simulink model "X_and_Y_position_calculator_of_the_center_of_mass_of_a_car"  (R2022b)
settings: Solver=VariableStepAuto  StartTime=0.0  StopTime=10.0  RelTol=1e-3
settings Model: Creator=tom  LastModifiedBy=tom

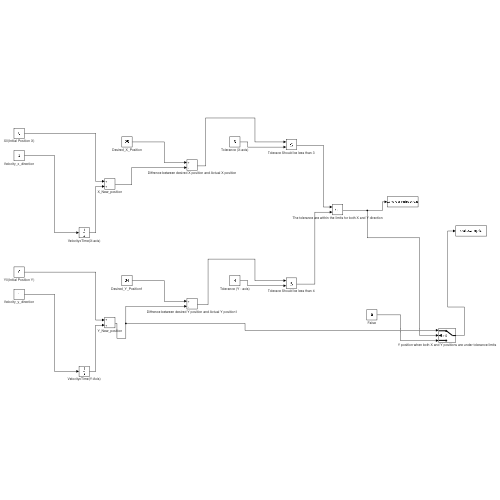
[thumbnail: Simulink's stored preview of the top-level diagram]
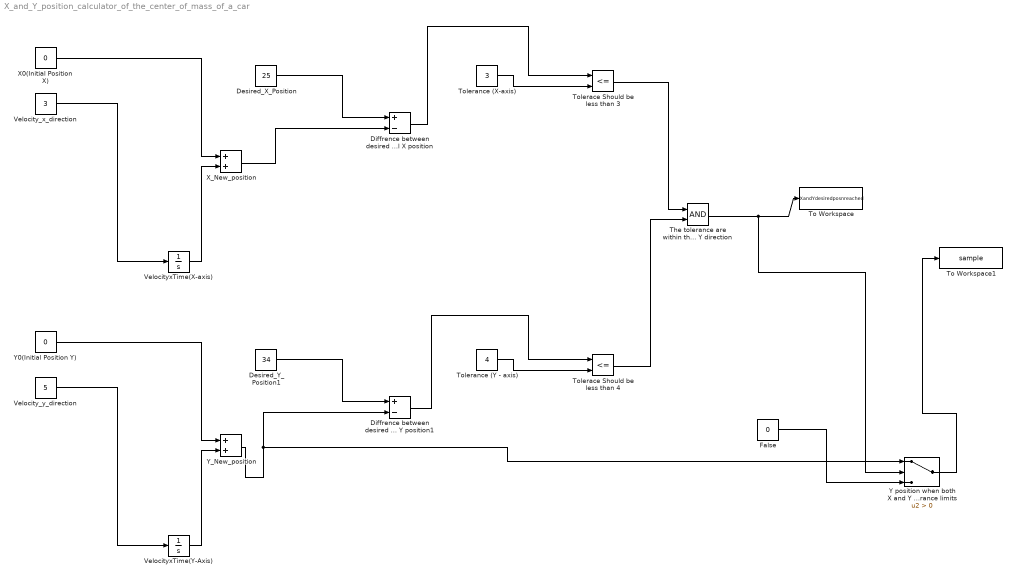
== system X_and_Y_position_calculator_of_the_center_of_mass_of_a_car ==
  Desired_X_Position : Constant  Value=25
  Desired_Y_Position1 : Constant  Value=34
  Diffrence between desired X position and Actual X position : Sum  Inputs=+-
  Diffrence between desired Y position and Actual Y position1 : Sum  Inputs=+-
  False : Constant  Value=0
  The tolerance are within the limits for both X and Y direction : Logic  AllPortsSameDT=off  OutDataTypeStr=boolean
  To Workspace : ToWorkspace  VariableName=XandYdesiredposnreached  SaveFormat=Timeseries  SampleTime=-1
  To Workspace1 : ToWorkspace  VariableName=sample  SaveFormat=Timeseries  SampleTime=-1
  Tolerace Should be less than 3 : RelationalOperator  Operator=<=  OutDataTypeStr=boolean  RndMeth=Simplest  InputSameDT=off
  Tolerace Should be less than 4 : RelationalOperator  Operator=<=  OutDataTypeStr=boolean  RndMeth=Simplest  InputSameDT=off
  Tolerance (X-axis) : Constant  Value=3
  Tolerance (Y - axis) : Constant  Value=4
  Velocity_x_direction : Constant  Value=3
  Velocity_y_direction : Constant  Value=5
  VelocityxTime(X-axis) : Integrator
  VelocityxTime(Y-Axis) : Integrator
  X0(Initial Position X) : Constant  Value=0
  X_New_position : Sum
  Y position when both X and Y positions are under tolerance limits : Switch  Criteria=u2 > Threshold  SaturateOnIntegerOverflow=off  InputSameDT=off
  Y0(Initial Position Y) : Constant  Value=0
  Y_New_position : Sum
  wires:
  X0(Initial Position X)/1 -> X_New_position/1
  Velocity_x_direction/1 -> VelocityxTime(X-axis)/1
  VelocityxTime(X-axis)/1 -> X_New_position/2
  Diffrence between desired X position and Actual X position/1 -> Tolerace Should be less than 3/1
  Tolerance (X-axis)/1 -> Tolerace Should be less than 3/2
  Desired_X_Position/1 -> Diffrence between desired X position and Actual X position/1
  X_New_position/1 -> Diffrence between desired X position and Actual X position/2
  Desired_Y_Position1/1 -> Diffrence between desired Y position and Actual Y position1/1
  Velocity_y_direction/1 -> VelocityxTime(Y-Axis)/1
  VelocityxTime(Y-Axis)/1 -> Y_New_position/2
  Y0(Initial Position Y)/1 -> Y_New_position/1
  Tolerance (Y - axis)/1 -> Tolerace Should be less than 4/2
  Tolerace Should be less than 3/1 -> The tolerance are within the limits for both X and Y direction/1
  Tolerace Should be less than 4/1 -> The tolerance are within the limits for both X and Y direction/2
  The tolerance are within the limits for both X and Y direction/1 -> Y position when both X and Y positions are under tolerance limits/2, To Workspace/1
  Y position when both X and Y positions are under tolerance limits/1 -> To Workspace1/1
  Diffrence between desired Y position and Actual Y position1/1 -> Tolerace Should be less than 4/1
  Y_New_position/1 -> Y position when both X and Y positions are under tolerance limits/1, Diffrence between desired Y position and Actual Y position1/2
  False/1 -> Y position when both X and Y positions are under tolerance limits/3
